simulink model "SAR_ADC_8Bit"  (R2016b)
settings: Solver=ode3  StartTime=0.0  StopTime=10.0  RelTol=1e-3  EnableMultiTasking=on
libraries: simulink_extras x34, simulink x22
settings Model: Creator=student  LastModifiedBy=Nahal
settings DataIOCC: LimitDataPoints=on  SaveFormat=Array  SignalLoggingSaveFormat=ModelDataLogs
settings OptimizationCC: InitFltsAndDblsToZero=on  LifeSpan=inf
settings DebuggingCC: SaveWithParameterizedLinksMsg=none  UnderspecifiedInitializationDetection=Classic  MergeDetectMultiDrivingBlocksExec=none  SignalResolutionControl=TryResolveAllWithWarning  SolverPrmCheckMsg=warning  MultiTaskDSMMsg=warning  MultiTaskCondExecSysMsg=none  FcnCallInpInsideContextMsg=warning  SFUnexpectedBacktrackingDiag=warning  SFNoUnconditionalDefaultTransitionDiag=warning  SFExecutionAtInitializationDiag=none
settings HardwareCC: ProdBitPerPointer=32  ProdBitPerSizeT=32  ProdBitPerPtrDiffT=32  ProdLargestAtomicFloat=None  ProdIntDivRoundTo=Undefined  ProdEndianess=Unspecified  ProdWordSize=32  ProdHWDeviceType=32-bit Generic
settings ModelReferenceCC: PropagateSignalLabelsOutOfModel=off
settings GRTTargetCC: TargetFcnLib=ansi_tfl_tmw.mat  TargetLangStandard=C89/C90 (ANSI)  CombineOutputUpdateFcns=off  GRTInterface=on
settings ConfigComp: CovMetricSettings=dw  CovHtmlReporting=on  CovSaveCumulativeToWorkspaceVar=on  CovSaveSingleToWorkspaceVar=on  CovExternalEMLEnable=off

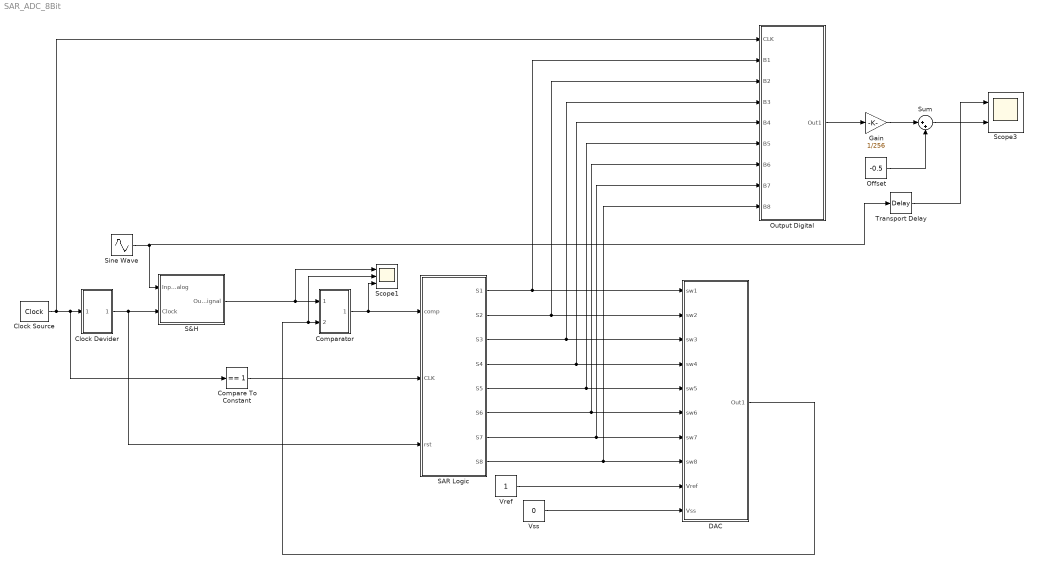
== system SAR_ADC_8Bit ==
  Clock Devider : Subsystem
  "Clock Source " : simulink_extras/Flip Flops/Clock  period=1/1000
  "Comparator " : Subsystem
  Compare To Constant : simulink/Logic and Bit Operations/Compare To Constant  relop===  const=1  OutDataTypeStr=boolean
  "DAC " : Subsystem
  Gain : Gain  Gain=1/256
  "Offset " : Constant  Value=-0.5
  "Output Digital " : Subsystem
  S&H : Subsystem
  "SAR Logic " : Subsystem
  Scope1 : Scope  NumInputPorts=3
  Scope3 : Scope  NumInputPorts=2
  Sine Wave : Sin  Amplitude=0.5  SampleTime=0
  Sum : Sum  Inputs=|++
  Transport Delay : TransportDelay  DelayTime=9/1000
  Vref : Constant
  Vss : Constant  Value=0
  wires:
  "Clock Source "/1 -> "Output Digital "/1("CLK "), Compare To Constant/1, Clock Devider/1(In1)
  Clock Devider/1(Out1) -> S&H/2(Clock), "SAR Logic "/3("rst ")
  Compare To Constant/1 -> "SAR Logic "/2("CLK ")
  Vref/1 -> "DAC "/9(Vref)
  Vss/1 -> "DAC "/10(Vss)
  "Comparator "/1(Out1) -> Scope1/3, "SAR Logic "/1(comp)
  "SAR Logic "/7(S7) -> "Output Digital "/8(B7), "DAC "/7(sw7)
  "SAR Logic "/8(S8) -> "Output Digital "/9(B8), "DAC "/8(sw8)
  "SAR Logic "/2(S2) -> "Output Digital "/3(B2), "DAC "/2(sw2)
  "SAR Logic "/5(S5) -> "Output Digital "/6(B5), "DAC "/5(sw5)
  "SAR Logic "/6(S6) -> "Output Digital "/7(B6), "DAC "/6(sw6)
  "SAR Logic "/3(S3) -> "Output Digital "/4(B3), "DAC "/3(sw3)
  "SAR Logic "/4(S4) -> "Output Digital "/5(B4), "DAC "/4(sw4)
  "SAR Logic "/1(S1) -> "Output Digital "/2(B1), "DAC "/1(sw1)
  "DAC "/1(Out1) -> Scope1/2, "Comparator "/2("inDAC ")
  S&H/1(Output Signal) -> Scope1/1, "Comparator "/1("Vin ")
  "Output Digital "/1(Out1) -> Gain/1
  Sine Wave/1 -> S&H/1("Input Analog "), Transport Delay/1
  Sum/1 -> Scope3/2
  "Offset "/1 -> Sum/2
  Gain/1 -> Sum/1
  Transport Delay/1 -> Scope3/1

== system SAR_ADC_8Bit/Clock Devider ==
  In1 : Inport
  Scope : Scope  NumInputPorts=2
  Subsystem : Subsystem
  Subsystem1 : Subsystem
  Subsystem2 : Subsystem
  Subsystem3 : Subsystem
  Out1 : Outport
  wires:
  In1/1 -> Subsystem2/1("CLK "), Scope/2
  Subsystem2/1(F/9) -> Scope/1, Out1/1

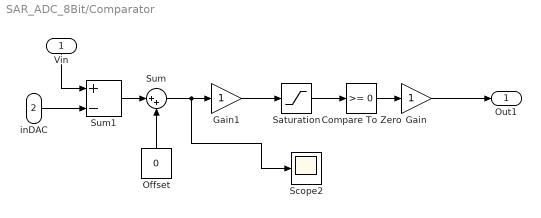
== system SAR_ADC_8Bit/Comparator  ==
  "Vin " : Inport
  "inDAC " : Inport  Port=2
  Compare To Zero : simulink/Logic and Bit Operations/Compare To Constant  relop=>=  const=0  OutDataTypeStr=boolean
  Gain : Gain
  Gain1 : Gain
  Offset : Constant  Value=0
  Saturation : Saturate  UpperLimit=1  LowerLimit=-1
  Scope2 : Scope
  Sum : Sum  Inputs=|++
  Sum1 : Sum  Inputs=+-
  Out1 : Outport
  wires:
  Gain/1 -> Out1/1
  Offset/1 -> Sum/2
  Sum/1 -> Scope2/1, Gain1/1
  Gain1/1 -> Saturation/1
  Saturation/1 -> Compare To Zero/1
  Compare To Zero/1 -> Gain/1
  "Vin "/1 -> Sum1/1
  "inDAC "/1 -> Sum1/2
  Sum1/1 -> Sum/1

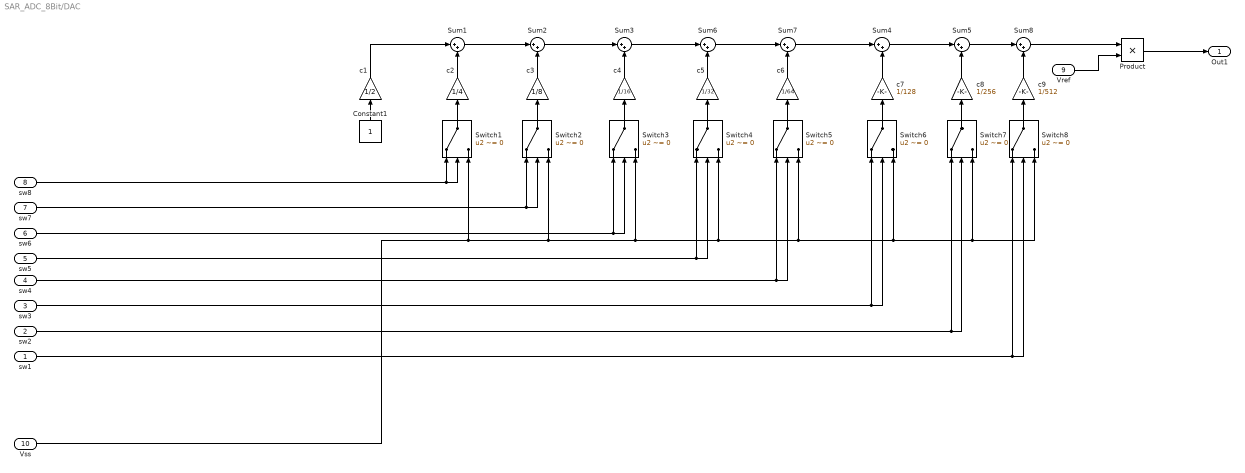
== system SAR_ADC_8Bit/DAC  ==
  sw1 : Inport
  sw2 : Inport  Port=2
  sw3 : Inport  Port=3
  sw4 : Inport  Port=4
  sw5 : Inport  Port=5
  sw6 : Inport  Port=6
  sw7 : Inport  Port=7
  sw8 : Inport  Port=8
  Vref : Inport  Port=9
  Vss : Inport  Port=10
  Constant1 : Constant
  Product : Product
  Sum{1..8} (8 alike) : Sum  Inputs=|++
  Switch{1..8} (8 alike) : Switch  Criteria=u2 ~= 0
  c1 : Gain  Gain=1/2
  c2 : Gain  Gain=1/4
  c3 : Gain  Gain=1/8
  c4 : Gain  Gain=1/16
  c5 : Gain  Gain=1/32
  c6 : Gain  Gain=1/64
  c7 : Gain  Gain=1/128
  c8 : Gain  Gain=1/256
  c9 : Gain  Gain=1/512
  Out1 : Outport
  wires:
  Sum4/1 -> Sum5/1
  c8/1 -> Sum5/2
  Switch6/1 -> c7/1
  Switch7/1 -> c8/1
  sw1/1 -> Switch8/1, Switch8/2
  sw4/1 -> Switch5/1, Switch5/2
  Switch1/1 -> c2/1
  Switch4/1 -> c5/1
  c6/1 -> Sum7/2
  Switch5/1 -> c6/1
  c7/1 -> Sum4/2
  Switch2/1 -> c3/1
  sw8/1 -> Switch1/2, Switch1/1
  Sum1/1 -> Sum2/1
  sw3/1 -> Switch6/1, Switch6/2
  c1/1 -> Sum1/1
  Sum6/1 -> Sum7/1
  c2/1 -> Sum1/2
  Sum3/1 -> Sum6/1
  c5/1 -> Sum6/2
  Sum7/1 -> Sum4/1
  c4/1 -> Sum3/2
  c3/1 -> Sum2/2
  Sum2/1 -> Sum3/1
  sw5/1 -> Switch4/1, Switch4/2
  Switch3/1 -> c4/1
  Product/1 -> Out1/1
  Vss/1 -> Switch3/3, Switch5/3, Switch6/3, Switch8/3, Switch7/3, Switch4/3, Switch2/3, Switch1/3
  sw2/1 -> Switch7/1, Switch7/2
  Constant1/1 -> c1/1
  sw7/1 -> Switch2/2, Switch2/1
  sw6/1 -> Switch3/1, Switch3/2
  Vref/1 -> Product/2
  c9/1 -> Sum8/2
  Switch8/1 -> c9/1
  Sum5/1 -> Sum8/1
  Sum8/1 -> Product/1

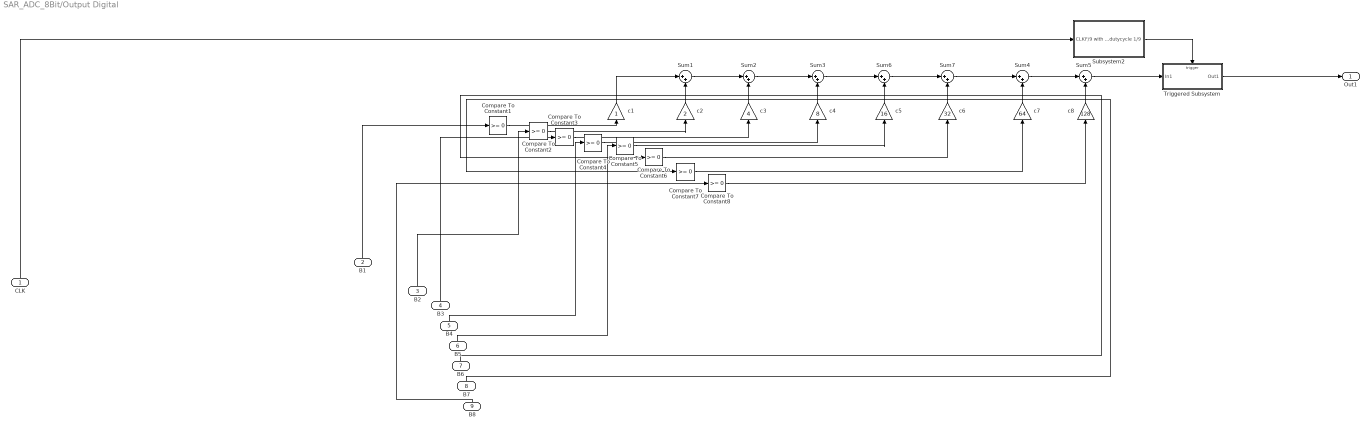
== system SAR_ADC_8Bit/Output Digital  ==
  "CLK " : Inport
  B1 : Inport  Port=2
  B2 : Inport  Port=3
  B3 : Inport  Port=4
  B4 : Inport  Port=5
  B5 : Inport  Port=6
  B6 : Inport  Port=7
  B7 : Inport  Port=8
  B8 : Inport  Port=9
  Compare To Constant{1..8} (8 alike) : simulink/Logic and Bit Operations/Compare To Constant  relop=>=  const=0  OutDataTypeStr=boolean
  Subsystem2 : Subsystem
  Sum{1..7} (7 alike) : Sum  Inputs=|++
  Triggered Subsystem : Subsystem  TreatAsAtomicUnit=on
  c1 : Gain
  c2 : Gain  Gain=2
  c3 : Gain  Gain=4
  c4 : Gain  Gain=8
  c5 : Gain  Gain=16
  c6 : Gain  Gain=32
  c7 : Gain  Gain=64
  c8 : Gain  Gain=128
  Out1 : Outport
  wires:
  Compare To Constant5/1 -> c5/1
  Compare To Constant4/1 -> c4/1
  Compare To Constant3/1 -> c3/1
  Compare To Constant7/1 -> c7/1
  Compare To Constant6/1 -> c6/1
  Triggered Subsystem/1(Out1) -> Out1/1
  Sum5/1 -> Triggered Subsystem/1(In1)
  c6/1 -> Sum7/2
  Sum1/1 -> Sum2/1
  Sum4/1 -> Sum5/1
  c1/1 -> Sum1/1
  Sum6/1 -> Sum7/1
  c2/1 -> Sum1/2
  c8/1 -> Sum5/2
  c7/1 -> Sum4/2
  Sum3/1 -> Sum6/1
  c3/1 -> Sum2/2
  c4/1 -> Sum3/2
  Sum7/1 -> Sum4/1
  c5/1 -> Sum6/2
  Sum2/1 -> Sum3/1
  Compare To Constant8/1 -> c8/1
  Compare To Constant2/1 -> c2/1
  Compare To Constant1/1 -> c1/1
  B5/1 -> Compare To Constant5/1
  B3/1 -> Compare To Constant3/1
  B2/1 -> Compare To Constant2/1
  "CLK "/1 -> Subsystem2/1("CLK ")
  B7/1 -> Compare To Constant7/1
  B6/1 -> Compare To Constant6/1
  B8/1 -> Compare To Constant8/1
  B1/1 -> Compare To Constant1/1
  B4/1 -> Compare To Constant4/1
  Subsystem2/1(F/9 with dutycycle 1/9) -> Triggered Subsystem/Trigger

== system SAR_ADC_8Bit/S&H ==
  "Input Analog " : Inport
  Clock : Inport  Port=2
  Constant : Constant  Value=0.5
  Gain : Gain  Gain=0
  Sum : Sum  Inputs=|++
  Sum2 : Sum  Inputs=|++
  Triggered Subsystem : Subsystem  TreatAsAtomicUnit=on
  Output Signal : Outport
  wires:
  Clock/1 -> Triggered Subsystem/Trigger
  Sum/1 -> Output Signal/1
  Gain/1 -> Sum/2
  Triggered Subsystem/1(Out1) -> Gain/1, Sum/1
  Sum2/1 -> Triggered Subsystem/1(In1)
  "Input Analog "/1 -> Sum2/1
  Constant/1 -> Sum2/2

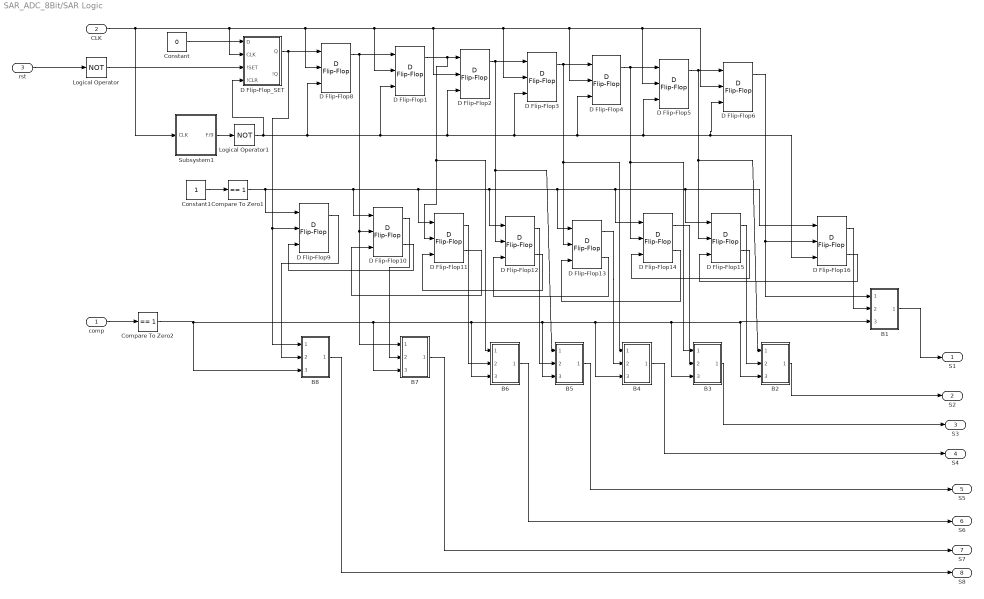
== system SAR_ADC_8Bit/SAR Logic  ==
  comp : Inport
  "CLK " : Inport  Port=2
  "rst " : Inport  Port=3
  B1 : Subsystem
  B2 : Subsystem
  B3 : Subsystem
  B4 : Subsystem
  B5 : Subsystem
  B6 : Subsystem
  B7 : Subsystem
  "B8 " : Subsystem
  Compare To Zero1 : simulink/Logic and Bit Operations/Compare To Constant  relop===  const=1  OutDataTypeStr=boolean
  Compare To Zero2 : simulink/Logic and Bit Operations/Compare To Constant  relop===  const=1  OutDataTypeStr=boolean
  Constant : Constant  Value=0
  Constant1 : Constant
  D Flip-Flop{1..6,8..16} (15 alike) : simulink_extras/Flip Flops/D Flip-Flop
  D Flip-Flop_SET : Subsystem
  Logical Operator : Logic  Operator=NOT  AllPortsSameDT=off  OutDataTypeStr=boolean
  Logical Operator1 : Logic  Operator=NOT  AllPortsSameDT=off  OutDataTypeStr=boolean
  Subsystem1 : Subsystem
  S1 : Outport
  S2 : Outport  Port=2
  S3 : Outport  Port=3
  S4 : Outport  Port=4
  S5 : Outport  Port=5
  S6 : Outport  Port=6
  S7 : Outport  Port=7
  S8 : Outport  Port=8
  wires:
  Constant/1 -> D Flip-Flop_SET/1(D)
  "CLK "/1 -> D Flip-Flop_SET/2(CLK), D Flip-Flop8/2, D Flip-Flop1/2, D Flip-Flop2/2, D Flip-Flop3/2, D Flip-Flop4/2, D Flip-Flop5/2, D Flip-Flop6/2, Subsystem1/1("CLK ")
  "rst "/1 -> Logical Operator/1
  D Flip-Flop2/1 -> D Flip-Flop3/1, B5/1(In1), D Flip-Flop12/2
  D Flip-Flop_SET/1(Q) -> D Flip-Flop9/2, "B8 "/1(In1), D Flip-Flop8/1
  Logical Operator/1 -> D Flip-Flop_SET/3(!SET)
  D Flip-Flop3/1 -> B4/1(In1), D Flip-Flop13/2, D Flip-Flop4/1
  Subsystem1/1(F/9) -> Logical Operator1/1
  D Flip-Flop11/2 -> D Flip-Flop10/3
  D Flip-Flop12/2 -> D Flip-Flop11/3
  D Flip-Flop13/2 -> D Flip-Flop12/3
  D Flip-Flop14/2 -> D Flip-Flop13/3
  D Flip-Flop15/2 -> D Flip-Flop14/3
  D Flip-Flop16/2 -> D Flip-Flop15/3
  Compare To Zero1/1 -> D Flip-Flop9/1, D Flip-Flop11/1, D Flip-Flop12/1, D Flip-Flop13/1, D Flip-Flop14/1, D Flip-Flop15/1, D Flip-Flop16/1, D Flip-Flop10/1
  D Flip-Flop10/2 -> D Flip-Flop9/3
  Constant1/1 -> Compare To Zero1/1
  comp/1 -> Compare To Zero2/1
  Compare To Zero2/1 -> "B8 "/3(In3), B6/3(In3), B1/3(In3), B2/3(In3), B3/3(In3), B4/3(In3), B5/3(In3), B7/3(In3)
  Logical Operator1/1 -> D Flip-Flop_SET/4("!CLR "), D Flip-Flop8/3, D Flip-Flop1/3, D Flip-Flop2/3, D Flip-Flop3/3, D Flip-Flop4/3, D Flip-Flop5/3, D Flip-Flop16/3, D Flip-Flop6/3
  D Flip-Flop1/1 -> B6/1(In1), D Flip-Flop11/2, D Flip-Flop2/1
  D Flip-Flop4/1 -> B3/1(In1), D Flip-Flop14/2, D Flip-Flop5/1
  D Flip-Flop5/1 -> B2/1(In1), D Flip-Flop15/2, D Flip-Flop6/1
  D Flip-Flop8/1 -> D Flip-Flop1/1, B7/1(In1), D Flip-Flop10/2
  D Flip-Flop16/1 -> B1/2(In2)
  B1/1(Out2) -> S1/1
  D Flip-Flop15/1 -> B2/2(In2)
  B2/1(Out2) -> S2/1
  D Flip-Flop14/1 -> B3/2(In2)
  B3/1(Out2) -> S3/1
  D Flip-Flop13/1 -> B4/2(In2)
  B4/1(Out2) -> S4/1
  D Flip-Flop12/1 -> B5/2(In2)
  B5/1(Out1) -> S5/1
  D Flip-Flop11/1 -> B6/2(In2)
  B6/1(Out1) -> S6/1
  D Flip-Flop10/1 -> B7/2(In2)
  D Flip-Flop9/1 -> "B8 "/2(In2)
  "B8 "/1(Out1) -> S8/1
  B7/1(Out1) -> S7/1
  D Flip-Flop6/1 -> D Flip-Flop16/2, B1/1(In1)

== system SAR_ADC_8Bit/Clock Devider/Subsystem ==
  "CLK " : Inport
  Constant1 : Constant
  D Flip-Flop4 : simulink_extras/Flip Flops/D Flip-Flop
  D Flip-Flop5 : simulink_extras/Flip Flops/D Flip-Flop
  D Flip-Flop6 : simulink_extras/Flip Flops/D Flip-Flop
  Logical Operator2 : Logic  Operator=OR  AllPortsSameDT=off  OutDataTypeStr=boolean
  Logical Operator4 : Logic  AllPortsSameDT=off  OutDataTypeStr=boolean
  Logical Operator5 : Logic  Operator=NOT  AllPortsSameDT=off  OutDataTypeStr=boolean
  F/3 : Outport
  wires:
  D Flip-Flop6/1 -> Logical Operator2/2
  D Flip-Flop4/2 -> Logical Operator4/1
  Constant1/1 -> D Flip-Flop6/3, D Flip-Flop5/3, D Flip-Flop4/3
  D Flip-Flop4/1 -> D Flip-Flop5/1
  Logical Operator4/1 -> D Flip-Flop4/1
  D Flip-Flop5/2 -> Logical Operator4/2
  "CLK "/1 -> Logical Operator5/1, D Flip-Flop5/2, D Flip-Flop4/2
  Logical Operator5/1 -> D Flip-Flop6/2
  Logical Operator2/1 -> F/3/1
  D Flip-Flop5/1 -> Logical Operator2/1, D Flip-Flop6/1

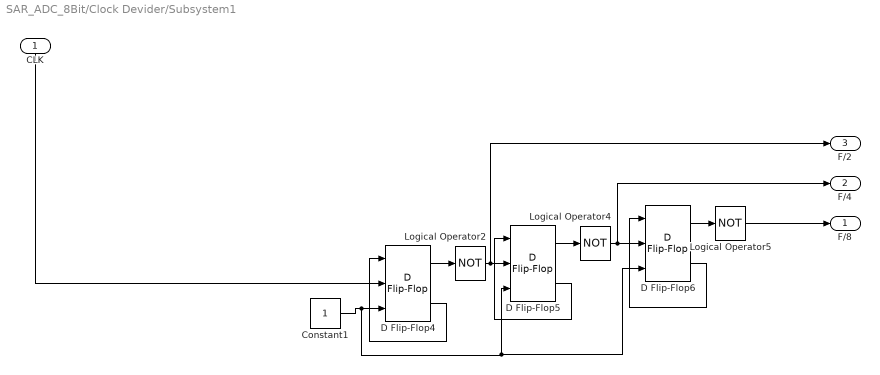
== system SAR_ADC_8Bit/Clock Devider/Subsystem1 ==
  "CLK " : Inport
  Constant1 : Constant
  D Flip-Flop4 : simulink_extras/Flip Flops/D Flip-Flop
  D Flip-Flop5 : simulink_extras/Flip Flops/D Flip-Flop
  D Flip-Flop6 : simulink_extras/Flip Flops/D Flip-Flop
  Logical Operator2 : Logic  Operator=NOT  AllPortsSameDT=off  OutDataTypeStr=boolean
  Logical Operator4 : Logic  Operator=NOT  AllPortsSameDT=off  OutDataTypeStr=boolean
  Logical Operator5 : Logic  Operator=NOT  AllPortsSameDT=off  OutDataTypeStr=boolean
  "F/8 " : Outport
  "F/4 " : Outport  Port=2
  "F/2 " : Outport  Port=3
  wires:
  D Flip-Flop4/2 -> D Flip-Flop4/1
  "CLK "/1 -> D Flip-Flop4/2
  Logical Operator5/1 -> "F/8 "/1
  D Flip-Flop5/1 -> Logical Operator4/1
  D Flip-Flop6/1 -> Logical Operator5/1
  Logical Operator4/1 -> "F/4 "/1, D Flip-Flop6/2
  Logical Operator2/1 -> "F/2 "/1, D Flip-Flop5/2
  D Flip-Flop5/2 -> D Flip-Flop5/1
  D Flip-Flop6/2 -> D Flip-Flop6/1
  Constant1/1 -> D Flip-Flop6/3, D Flip-Flop5/3, D Flip-Flop4/3
  D Flip-Flop4/1 -> Logical Operator2/1

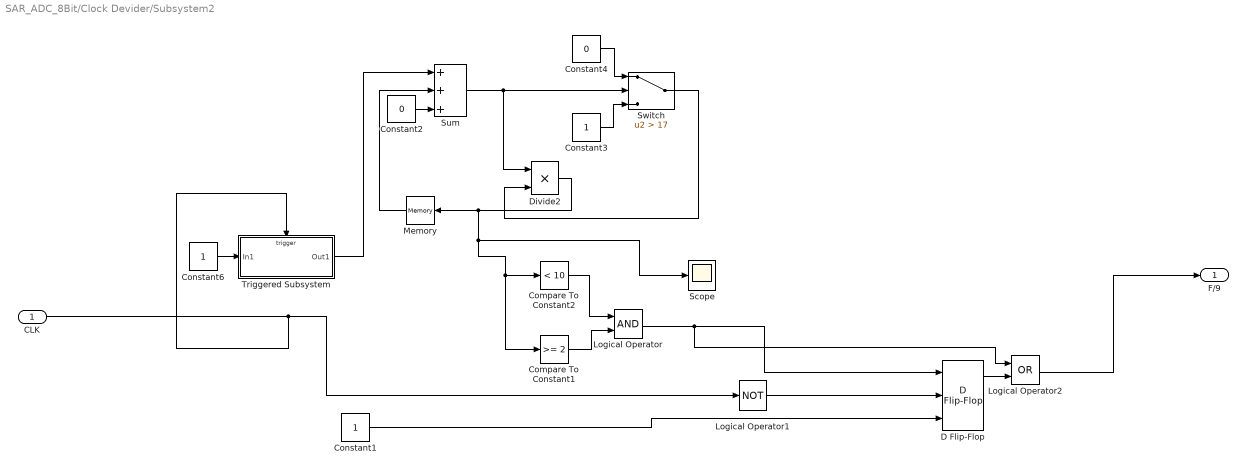
== system SAR_ADC_8Bit/Clock Devider/Subsystem2 ==
  "CLK " : Inport
  Compare To Constant1 : simulink/Logic and Bit Operations/Compare To Constant  relop=>=  const=2  OutDataTypeStr=boolean
  Compare To Constant2 : simulink/Logic and Bit Operations/Compare To Constant  relop=<  const=10  OutDataTypeStr=boolean
  Constant1 : Constant
  Constant2 : Constant  Value=0
  Constant3 : Constant
  Constant4 : Constant  Value=0
  Constant6 : Constant
  D Flip-Flop : simulink_extras/Flip Flops/D Flip-Flop
  Divide2 : Product
  Logical Operator : Logic  AllPortsSameDT=off  OutDataTypeStr=boolean
  Logical Operator1 : Logic  Operator=NOT  AllPortsSameDT=off  OutDataTypeStr=boolean
  Logical Operator2 : Logic  Operator=OR  AllPortsSameDT=off  OutDataTypeStr=boolean
  Memory : Memory
  Scope : Scope
  Sum : Sum  Inputs=3
  Switch : Switch  Criteria=u2 > Threshold  Threshold=17
  Triggered Subsystem : Subsystem  TreatAsAtomicUnit=on
  F/9 : Outport
  wires:
  Sum/1 -> Divide2/1, Switch/2
  Memory/1 -> Sum/2
  Triggered Subsystem/1(Out1) -> Sum/1
  Constant1/1 -> D Flip-Flop/3
  Compare To Constant2/1 -> Logical Operator/1
  Logical Operator1/1 -> D Flip-Flop/2
  Logical Operator/1 -> Logical Operator2/1, D Flip-Flop/1
  D Flip-Flop/1 -> Logical Operator2/2
  Logical Operator2/1 -> F/9/1
  Switch/1 -> Divide2/2
  Constant4/1 -> Switch/1
  Constant3/1 -> Switch/3
  Compare To Constant1/1 -> Logical Operator/2
  Divide2/1 -> Scope/1, Compare To Constant1/1, Compare To Constant2/1, Memory/1
  Constant6/1 -> Triggered Subsystem/1(In1)
  "CLK "/1 -> Triggered Subsystem/Trigger, Logical Operator1/1
  Constant2/1 -> Sum/3

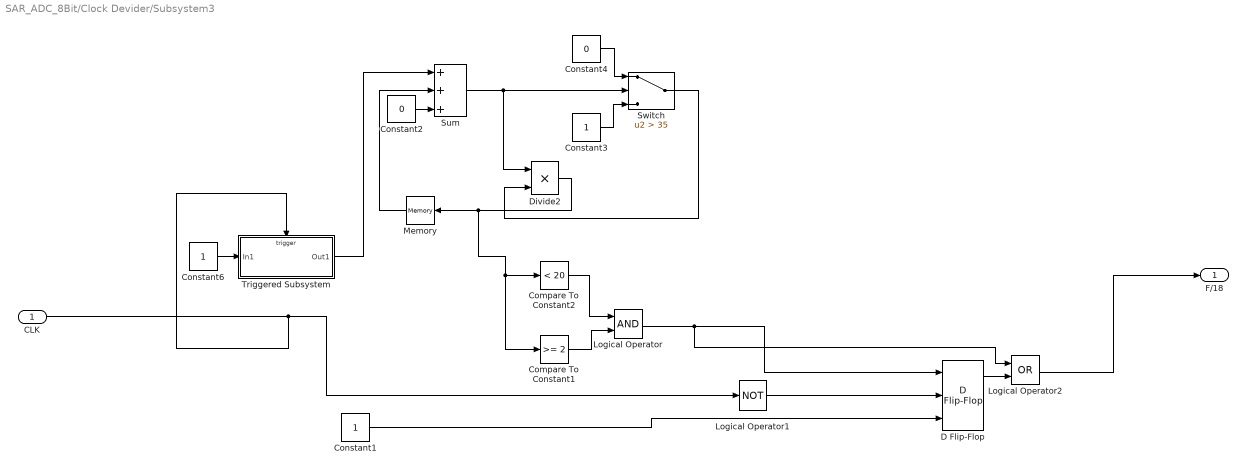
== system SAR_ADC_8Bit/Clock Devider/Subsystem3 ==
  "CLK " : Inport
  Compare To Constant1 : simulink/Logic and Bit Operations/Compare To Constant  relop=>=  const=2  OutDataTypeStr=boolean
  Compare To Constant2 : simulink/Logic and Bit Operations/Compare To Constant  relop=<  const=20  OutDataTypeStr=boolean
  Constant1 : Constant
  Constant2 : Constant  Value=0
  Constant3 : Constant
  Constant4 : Constant  Value=0
  Constant6 : Constant
  D Flip-Flop : simulink_extras/Flip Flops/D Flip-Flop
  Divide2 : Product
  Logical Operator : Logic  AllPortsSameDT=off  OutDataTypeStr=boolean
  Logical Operator1 : Logic  Operator=NOT  AllPortsSameDT=off  OutDataTypeStr=boolean
  Logical Operator2 : Logic  Operator=OR  AllPortsSameDT=off  OutDataTypeStr=boolean
  Memory : Memory
  Sum : Sum  Inputs=3
  Switch : Switch  Criteria=u2 > Threshold  Threshold=35
  Triggered Subsystem : Subsystem  TreatAsAtomicUnit=on
  "F/18 " : Outport
  wires:
  Constant2/1 -> Sum/3
  "CLK "/1 -> Logical Operator1/1, Triggered Subsystem/Trigger
  Constant6/1 -> Triggered Subsystem/1(In1)
  Divide2/1 -> Memory/1, Compare To Constant2/1, Compare To Constant1/1
  Compare To Constant1/1 -> Logical Operator/2
  Constant3/1 -> Switch/3
  Constant4/1 -> Switch/1
  Switch/1 -> Divide2/2
  Logical Operator2/1 -> "F/18 "/1
  D Flip-Flop/1 -> Logical Operator2/2
  Logical Operator/1 -> D Flip-Flop/1, Logical Operator2/1
  Logical Operator1/1 -> D Flip-Flop/2
  Compare To Constant2/1 -> Logical Operator/1
  Constant1/1 -> D Flip-Flop/3
  Triggered Subsystem/1(Out1) -> Sum/1
  Memory/1 -> Sum/2
  Sum/1 -> Switch/2, Divide2/1

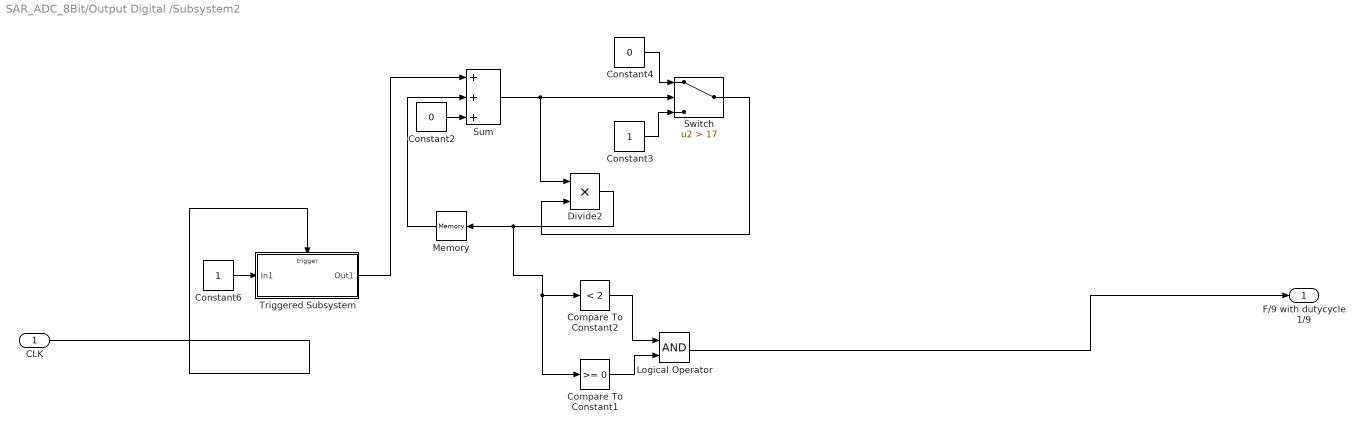
== system SAR_ADC_8Bit/Output Digital /Subsystem2 ==
  "CLK " : Inport
  Compare To Constant1 : simulink/Logic and Bit Operations/Compare To Constant  relop=>=  const=0  OutDataTypeStr=boolean
  Compare To Constant2 : simulink/Logic and Bit Operations/Compare To Constant  relop=<  const=2  OutDataTypeStr=boolean
  Constant2 : Constant  Value=0
  Constant3 : Constant
  Constant4 : Constant  Value=0
  Constant6 : Constant
  Divide2 : Product
  Logical Operator : Logic  AllPortsSameDT=off  OutDataTypeStr=boolean
  Memory : Memory
  Sum : Sum  Inputs=3
  Switch : Switch  Criteria=u2 > Threshold  Threshold=17
  Triggered Subsystem : Subsystem  TreatAsAtomicUnit=on
  F/9 with dutycycle 1/9 : Outport
  wires:
  Sum/1 -> Divide2/1, Switch/2
  Memory/1 -> Sum/2
  Triggered Subsystem/1(Out1) -> Sum/1
  Compare To Constant2/1 -> Logical Operator/1
  Logical Operator/1 -> F/9 with dutycycle 1/9/1
  Switch/1 -> Divide2/2
  Constant4/1 -> Switch/1
  Constant3/1 -> Switch/3
  Compare To Constant1/1 -> Logical Operator/2
  Divide2/1 -> Compare To Constant1/1, Compare To Constant2/1, Memory/1
  Constant6/1 -> Triggered Subsystem/1(In1)
  "CLK "/1 -> Triggered Subsystem/Trigger
  Constant2/1 -> Sum/3

== system SAR_ADC_8Bit/Output Digital /Triggered Subsystem ==
  In1 : Inport
  Trigger : TriggerPort  VariantControl=Variant
  Out1 : Outport
  wires:
  In1/1 -> Out1/1

== system SAR_ADC_8Bit/S&H/Triggered Subsystem ==
  In1 : Inport
  Trigger : TriggerPort  VariantControl=Variant
  Out1 : Outport
  wires:
  In1/1 -> Out1/1

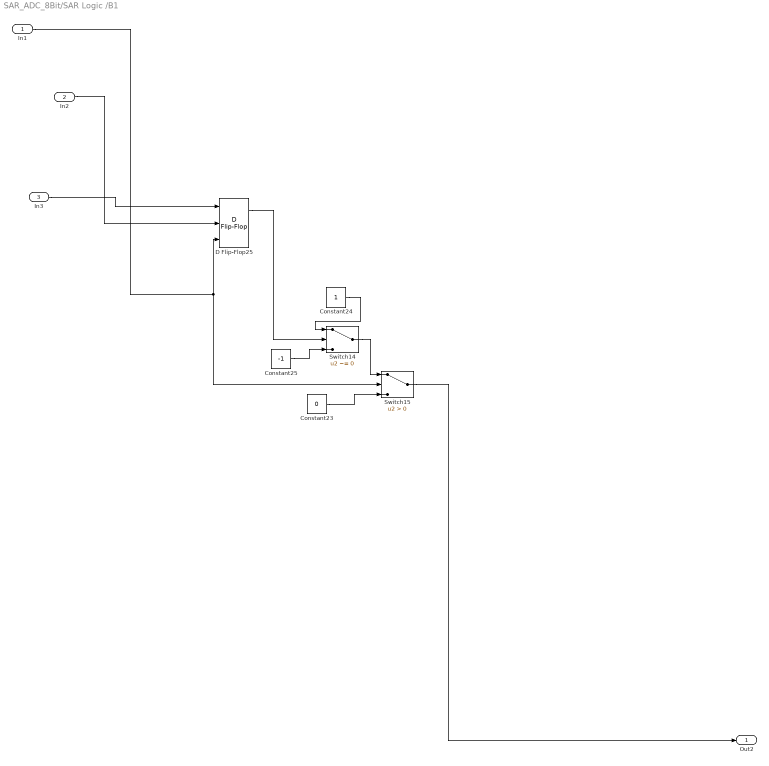
== system SAR_ADC_8Bit/SAR Logic /B1 ==
  In1 : Inport
  In2 : Inport  Port=2
  In3 : Inport  Port=3
  Constant23 : Constant  Value=0
  Constant24 : Constant
  Constant25 : Constant  Value=-1
  D Flip-Flop25 : simulink_extras/Flip Flops/D Flip-Flop
  Switch14 : Switch  Criteria=u2 ~= 0
  Switch15 : Switch  Criteria=u2 > Threshold
  Out2 : Outport
  wires:
  In3/1 -> D Flip-Flop25/1
  In1/1 -> Switch15/2, D Flip-Flop25/3
  In2/1 -> D Flip-Flop25/2
  Switch14/1 -> Switch15/1
  Constant23/1 -> Switch15/3
  D Flip-Flop25/1 -> Switch14/2
  Switch15/1 -> Out2/1
  Constant24/1 -> Switch14/1
  Constant25/1 -> Switch14/3

== system SAR_ADC_8Bit/SAR Logic /B2 ==
  In1 : Inport
  In2 : Inport  Port=2
  In3 : Inport  Port=3
  Constant20 : Constant  Value=0
  Constant21 : Constant
  Constant22 : Constant  Value=-1
  D Flip-Flop24 : simulink_extras/Flip Flops/D Flip-Flop
  Switch12 : Switch  Criteria=u2 ~= 0
  Switch13 : Switch  Criteria=u2 > Threshold
  Out2 : Outport
  wires:
  Constant21/1 -> Switch12/1
  Switch12/1 -> Switch13/1
  D Flip-Flop24/1 -> Switch12/2
  Constant20/1 -> Switch13/3
  Constant22/1 -> Switch12/3
  Switch13/1 -> Out2/1
  In2/1 -> D Flip-Flop24/2
  In3/1 -> D Flip-Flop24/1
  In1/1 -> Switch13/2, D Flip-Flop24/3

== system SAR_ADC_8Bit/SAR Logic /B3 ==
  In1 : Inport
  In2 : Inport  Port=2
  In3 : Inport  Port=3
  Constant17 : Constant  Value=0
  Constant18 : Constant
  Constant19 : Constant  Value=-1
  D Flip-Flop23 : simulink_extras/Flip Flops/D Flip-Flop
  Switch10 : Switch  Criteria=u2 ~= 0
  Switch11 : Switch  Criteria=u2 > Threshold
  Out2 : Outport
  wires:
  D Flip-Flop23/1 -> Switch10/2
  In3/1 -> D Flip-Flop23/1
  In1/1 -> Switch11/2, D Flip-Flop23/3
  Switch10/1 -> Switch11/1
  Constant19/1 -> Switch10/3
  Constant18/1 -> Switch10/1
  Constant17/1 -> Switch11/3
  Switch11/1 -> Out2/1
  In2/1 -> D Flip-Flop23/2

== system SAR_ADC_8Bit/SAR Logic /B4 ==
  In1 : Inport
  In2 : Inport  Port=2
  In3 : Inport  Port=3
  Constant14 : Constant  Value=0
  Constant15 : Constant
  Constant16 : Constant  Value=-1
  D Flip-Flop22 : simulink_extras/Flip Flops/D Flip-Flop
  Switch8 : Switch  Criteria=u2 ~= 0
  Switch9 : Switch  Criteria=u2 > Threshold
  Out2 : Outport
  wires:
  In1/1 -> D Flip-Flop22/3, Switch9/2
  In3/1 -> D Flip-Flop22/1
  Switch9/1 -> Out2/1
  In2/1 -> D Flip-Flop22/2
  D Flip-Flop22/1 -> Switch8/2
  Constant15/1 -> Switch8/1
  Switch8/1 -> Switch9/1
  Constant16/1 -> Switch8/3
  Constant14/1 -> Switch9/3

== system SAR_ADC_8Bit/SAR Logic /B5 ==
  In1 : Inport
  In2 : Inport  Port=2
  In3 : Inport  Port=3
  Constant11 : Constant  Value=0
  Constant12 : Constant
  Constant13 : Constant  Value=-1
  D Flip-Flop21 : simulink_extras/Flip Flops/D Flip-Flop
  Switch6 : Switch  Criteria=u2 ~= 0
  Switch7 : Switch  Criteria=u2 > Threshold
  Out1 : Outport
  wires:
  Constant12/1 -> Switch6/1
  Switch6/1 -> Switch7/1
  Constant13/1 -> Switch6/3
  Constant11/1 -> Switch7/3
  D Flip-Flop21/1 -> Switch6/2
  Switch7/1 -> Out1/1
  In1/1 -> Switch7/2, D Flip-Flop21/3
  In3/1 -> D Flip-Flop21/1
  In2/1 -> D Flip-Flop21/2

== system SAR_ADC_8Bit/SAR Logic /B6 ==
  In1 : Inport
  In2 : Inport  Port=2
  In3 : Inport  Port=3
  Constant10 : Constant  Value=0
  Constant8 : Constant
  Constant9 : Constant  Value=-1
  D Flip-Flop20 : simulink_extras/Flip Flops/D Flip-Flop
  Switch4 : Switch  Criteria=u2 ~= 0
  Switch5 : Switch  Criteria=u2 > Threshold
  Out1 : Outport
  wires:
  D Flip-Flop20/1 -> Switch4/2
  In1/1 -> Switch5/2, D Flip-Flop20/3
  In3/1 -> D Flip-Flop20/1
  Switch5/1 -> Out1/1
  In2/1 -> D Flip-Flop20/2
  Switch4/1 -> Switch5/1
  Constant8/1 -> Switch4/1
  Constant10/1 -> Switch5/3
  Constant9/1 -> Switch4/3

== system SAR_ADC_8Bit/SAR Logic /B7 ==
  In1 : Inport
  In2 : Inport  Port=2
  In3 : Inport  Port=3
  Constant5 : Constant
  Constant6 : Constant  Value=-1
  Constant7 : Constant  Value=0
  D Flip-Flop19 : simulink_extras/Flip Flops/D Flip-Flop
  Switch2 : Switch  Criteria=u2 ~= 0
  Switch3 : Switch  Criteria=u2 > Threshold
  Out1 : Outport
  wires:
  Switch3/1 -> Out1/1
  In1/1 -> Switch3/2, D Flip-Flop19/3
  In3/1 -> D Flip-Flop19/1
  D Flip-Flop19/1 -> Switch2/2
  Switch2/1 -> Switch3/1
  Constant7/1 -> Switch3/3
  Constant5/1 -> Switch2/1
  Constant6/1 -> Switch2/3
  In2/1 -> D Flip-Flop19/2

== system SAR_ADC_8Bit/SAR Logic /B8  ==
  In1 : Inport
  In2 : Inport  Port=2
  In3 : Inport  Port=3
  Constant2 : Constant
  Constant3 : Constant  Value=-1
  Constant4 : Constant  Value=0
  D Flip-Flop18 : simulink_extras/Flip Flops/D Flip-Flop
  Switch : Switch  Criteria=u2 ~= 0
  Switch1 : Switch  Criteria=u2 > Threshold
  Out1 : Outport
  wires:
  Switch1/1 -> Out1/1
  In3/1 -> D Flip-Flop18/1
  In1/1 -> Switch1/2, D Flip-Flop18/3
  Constant2/1 -> Switch/1
  Constant3/1 -> Switch/3
  D Flip-Flop18/1 -> Switch/2
  In2/1 -> D Flip-Flop18/2
  Switch/1 -> Switch1/1
  Constant4/1 -> Switch1/3

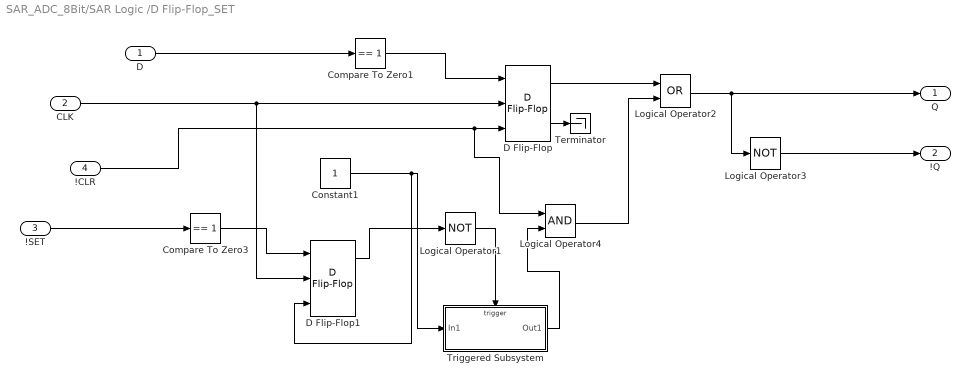
== system SAR_ADC_8Bit/SAR Logic /D Flip-Flop_SET ==
  D : Inport
  CLK : Inport  Port=2
  !SET : Inport  Port=3
  "!CLR " : Inport  Port=4
  Compare To Zero1 : simulink/Logic and Bit Operations/Compare To Constant  relop===  const=1  OutDataTypeStr=boolean
  Compare To Zero3 : simulink/Logic and Bit Operations/Compare To Constant  relop===  const=1  OutDataTypeStr=boolean
  Constant1 : Constant
  D Flip-Flop : simulink_extras/Flip Flops/D Flip-Flop
  D Flip-Flop1 : simulink_extras/Flip Flops/D Flip-Flop
  Logical Operator1 : Logic  Operator=NOT  AllPortsSameDT=off  OutDataTypeStr=boolean
  Logical Operator2 : Logic  Operator=OR  AllPortsSameDT=off  OutDataTypeStr=boolean
  Logical Operator3 : Logic  Operator=NOT  AllPortsSameDT=off  OutDataTypeStr=boolean
  Logical Operator4 : Logic  AllPortsSameDT=off  OutDataTypeStr=boolean
  Terminator : Terminator
  Triggered Subsystem : Subsystem  TreatAsAtomicUnit=on
  Q : Outport
  !Q : Outport  Port=2
  wires:
  D Flip-Flop/1 -> Logical Operator2/1
  Logical Operator4/1 -> Logical Operator2/2
  Compare To Zero1/1 -> D Flip-Flop/1
  !SET/1 -> Compare To Zero3/1
  D/1 -> Compare To Zero1/1
  D Flip-Flop/2 -> Terminator/1
  CLK/1 -> D Flip-Flop1/2, D Flip-Flop/2
  Logical Operator2/1 -> Logical Operator3/1, Q/1
  Logical Operator3/1 -> !Q/1
  Logical Operator1/1 -> Triggered Subsystem/Trigger
  Triggered Subsystem/1(Out1) -> Logical Operator4/2
  Compare To Zero3/1 -> D Flip-Flop1/1
  D Flip-Flop1/1 -> Logical Operator1/1
  Constant1/1 -> D Flip-Flop1/3, Triggered Subsystem/1(In1)
  "!CLR "/1 -> Logical Operator4/1, D Flip-Flop/3

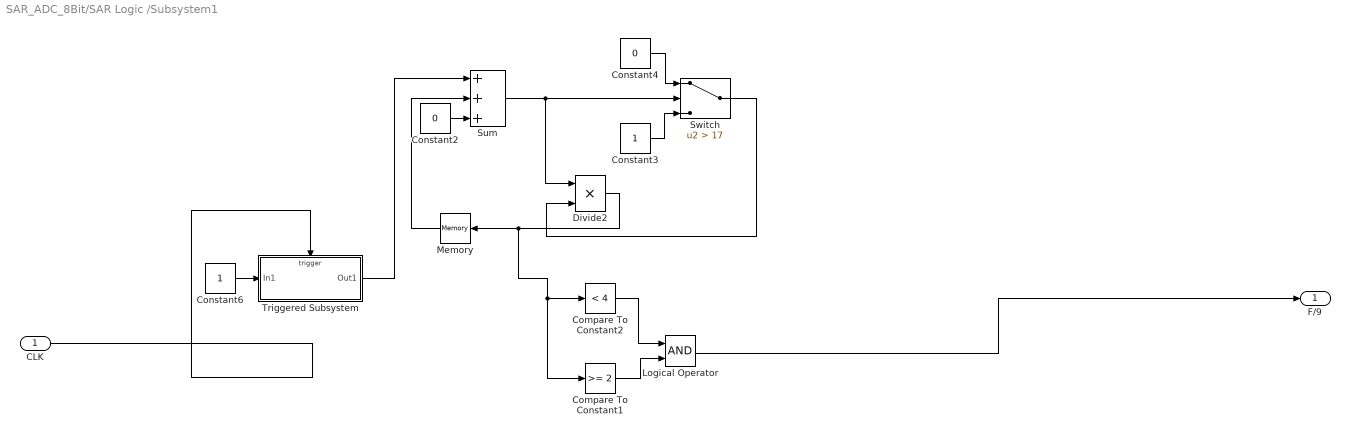
== system SAR_ADC_8Bit/SAR Logic /Subsystem1 ==
  "CLK " : Inport
  Compare To Constant1 : simulink/Logic and Bit Operations/Compare To Constant  relop=>=  const=2  OutDataTypeStr=boolean
  Compare To Constant2 : simulink/Logic and Bit Operations/Compare To Constant  relop=<  const=4  OutDataTypeStr=boolean
  Constant2 : Constant  Value=0
  Constant3 : Constant
  Constant4 : Constant  Value=0
  Constant6 : Constant
  Divide2 : Product
  Logical Operator : Logic  AllPortsSameDT=off  OutDataTypeStr=boolean
  Memory : Memory
  Sum : Sum  Inputs=3
  Switch : Switch  Criteria=u2 > Threshold  Threshold=17
  Triggered Subsystem : Subsystem  TreatAsAtomicUnit=on
  F/9 : Outport
  wires:
  Sum/1 -> Divide2/1, Switch/2
  Memory/1 -> Sum/2
  Triggered Subsystem/1(Out1) -> Sum/1
  Compare To Constant2/1 -> Logical Operator/1
  "CLK "/1 -> Triggered Subsystem/Trigger
  Logical Operator/1 -> F/9/1
  Switch/1 -> Divide2/2
  Constant4/1 -> Switch/1
  Constant3/1 -> Switch/3
  Compare To Constant1/1 -> Logical Operator/2
  Divide2/1 -> Compare To Constant1/1, Compare To Constant2/1, Memory/1
  Constant6/1 -> Triggered Subsystem/1(In1)
  Constant2/1 -> Sum/3

== system SAR_ADC_8Bit/Clock Devider/Subsystem2/Triggered Subsystem ==
  In1 : Inport
  Trigger : TriggerPort  TriggerType=falling  VariantControl=Variant
  Out1 : Outport
  wires:
  In1/1 -> Out1/1

== system SAR_ADC_8Bit/Clock Devider/Subsystem3/Triggered Subsystem ==
  In1 : Inport
  Trigger : TriggerPort  TriggerType=falling  VariantControl=Variant
  Out1 : Outport
  wires:
  In1/1 -> Out1/1

== system SAR_ADC_8Bit/Output Digital /Subsystem2/Triggered Subsystem ==
  In1 : Inport
  Trigger : TriggerPort  TriggerType=falling  VariantControl=Variant
  Out1 : Outport
  wires:
  In1/1 -> Out1/1

== system SAR_ADC_8Bit/SAR Logic /D Flip-Flop_SET/Triggered Subsystem ==
  In1 : Inport
  Trigger : TriggerPort  VariantControl=Variant
  Out1 : Outport
  wires:
  In1/1 -> Out1/1

== system SAR_ADC_8Bit/SAR Logic /Subsystem1/Triggered Subsystem ==
  In1 : Inport
  Trigger : TriggerPort  TriggerType=falling  VariantControl=Variant
  Out1 : Outport
  wires:
  In1/1 -> Out1/1
